simulink model "TP2_Sim"  (R2024b)
settings: Solver=VariableStepAuto  StartTime=0.0  StopTime=100.0  RelTol=1e-3
StopFcn:
  | x = out.X;
  | plot3(x(1,:), x(2,:), x(3,:));
  | grid on;
settings Model: Creator=user  LastModifiedBy=user

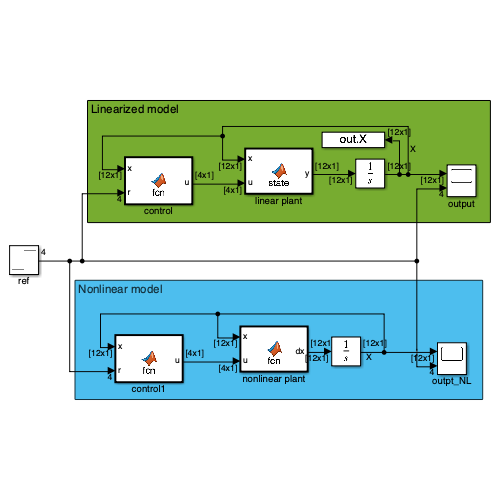
[thumbnail: Simulink's stored preview of the top-level diagram]
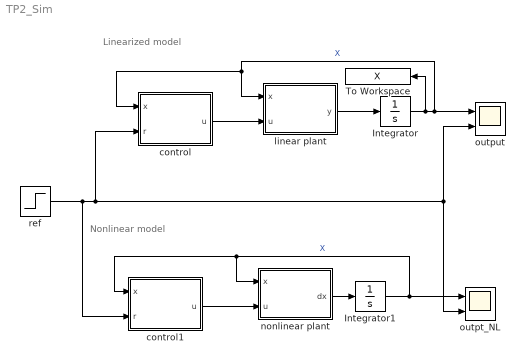
== system TP2_Sim ==
  note: Nonlinear model
  note: Linearized model
  Integrator : Integrator  InitialCondition=0.0*[1 1 1 1 1 1 1 1 1 1 1 1]'
  Integrator1 : Integrator  InitialCondition=0.0*[1 1 1 1 1 1 1 1 1 1 1 1]'
  To Workspace : ToWorkspace  VariableName=X  SampleTime=-1
  control : MATLAB Function  TreatAsAtomicUnit=on
  control1 : MATLAB Function  TreatAsAtomicUnit=on
  linear plant : MATLAB Function  TreatAsAtomicUnit=on
  nonlinear plant : MATLAB Function  TreatAsAtomicUnit=on
  outpt_NL : Scope  NumInputPorts=2
  output : Scope  NumInputPorts=2
  ref : Step  After=[2, 0, 0, 1]'  SampleTime=0
  wires:
  Integrator/1 -> To Workspace/1, control/1(x), linear plant/1(x), output/1  "X"
  control/1(u) -> linear plant/2(u)
  linear plant/1(y) -> Integrator/1
  ref/1 -> output/2, outpt_NL/2, control/2(r), control1/2(r)
  nonlinear plant/1(dx) -> Integrator1/1
  Integrator1/1 -> control1/1(x), nonlinear plant/1(x), outpt_NL/1  "X"
  control1/1(u) -> nonlinear plant/2(u)

== matlab function TP2_Sim/linear plant ==
  data: x input; u input; y output
function y = state(x, u)
% Define the state derivatives
% x(1) = x7, x(2) = x8, ..., x(6) = x12

% Constants
m = 1.62;
Izz = 0.026;
Iyy = 0.01667;
Ixx = 0.0184;
g = 9.81;

% Inputs
u1 = u(1);
u2 = u(2);
u3 = u(3);
u4 = u(4);

% State variables
phi = x(4);  % Roll angle
theta = x(5); % Pitch angle
psi = x(6);   % Yaw angle

% Dynamics equations
dx = zeros(12, 1);
dx(1) = x(7);
dx(2) = x(8);
dx(3) = x(9);
dx(4) = x(10);
dx(5) = x(11);
dx(6) = x(12);
dx(7) = (cos(x(6)) * x(5) + x(4) * sin(x(6))) * u1 / m;
dx(8) = (-cos(x(6)) * x(4) + x(5) * sin(x(6))) * u1 / m;
dx(9) = u1/m - g;
dx(10) = u2 / Ixx;
dx(11) = u3 / Iyy;
dx(12) = u4 / Izz;
y = dx;
end

== matlab function TP2_Sim/nonlinear plant ==
  data: x input; u input; dx output
function dx = fcn(x,u)
g  = 9.81;
m = 1.62; 
Ixx = 0.01184;
Iyy = 0.01667;
Izz = 0.026; 

dx = zeros(12,1);
dx(1) = x(7);
dx(2) = x(8);
dx(3) = x(9);
dx(4) = x(10);
dx(5) = x(11);
dx(6) = x(12);
dx(7) = (cos(x(4))*cos(x(6))*sin(x(5)) + sin(x(4)*sin(x(5)))*(u(1)/m));
dx(8) = (-cos(x(6))*sin(x(4)) + cos(x(4))*sin(x(6))*sin(x(5)))*(u(1)/m);
dx(9) = -g + cos(x(4))*cos(x(5))*(u(1)/m);
dx(10) = 1/Ixx*(x(11)*x(12)*(Iyy-Izz) + u(2));
dx(11) = 1/Iyy*(x(10)*x(12)*(-Ixx + Izz) + u(3));
dx(12) = 1/Izz*(x(10)*x(11)*(Ixx - Izz) + u(4));

== matlab function TP2_Sim/control1 ==
  data: x input; u output; r input; K parameter
function u = fcn(x, r, K)
% r - reference input for z, phi, and theta
m = 1.62;
g = 9.81;
u = zeros(4,1);
u(1) = (K(1)*(r(1)-x(3)) - K(2)*x(9) + g)*m;
u(2) = K(1)*(r(2)-x(4)) - K(2)*x(10);
u(3) = K(1)*(r(3)-x(5)) - K(2)*x(11);
u(4) = K(1)*(r(4)-x(6)) - K(2)*x(12);

== matlab function TP2_Sim/control ==
  data: x input; u output; r input; K parameter
function u = fcn(x, r, K)
% r - reference input for z, phi, and theta
k1 = 5;
k2 = 4;
m = 1.62;
g = 9.81;
u = zeros(4,1);
% u(1) = 1;
u(1) = (K(1)*(r(1)-x(3)) - K(2)*x(9) + g)*m;
u(2) = K(1)*(r(2)-x(4)) - K(2)*x(10);
u(3) = K(1)*(r(3)-x(5)) - K(2)*x(11);
u(4) = K(1)*(r(4)-x(6)) - K(2)*x(12);
